simulink model "lane_departure"  (R2017a)
settings: Solver=FixedStepDiscrete  StartTime=0.0  StopTime=inf  FixedStep=1/25  RelTol=1e-3  EnableMultiTasking=on
libraries: visionsinks x1, dspvision x1, embdlinuxlib x1
settings Model: SimulationMode=external  Creator=ChiChaChai  LastModifiedBy=ChiChaChai
settings SolverCC: PositivePriorityOrder=on  AutoInsertRateTranBlk=on
settings OptimizationCC: UseFloatMulNetSlope=on  PassReuseOutputArgsAs=Individual arguments  ZeroExternalMemoryAtStartup=off  ZeroInternalMemoryAtStartup=off  NoFixptDivByZeroProtection=on  EfficientFloat2IntCast=on  LifeSpan=1  MaxStackSize=64
settings DebuggingCC: ParameterTunabilityLossMsg=error
settings HardwareCC: ProdBitPerPointer=32  ProdBitPerSizeT=32  ProdBitPerPtrDiffT=32  ProdLargestAtomicInteger=Long  ProdLargestAtomicFloat=Double  ProdWordSize=32  ProdHWDeviceType=ARM Compatible->ARM Cortex
settings SFSimCC: MATLABDynamicMemAlloc=off
settings RTWCC: SystemTargetFile=ert.tlc  HardwareBoard=Raspberry Pi  TLCOptions="-aInlineSetEventsForThisBaseRateFcn=TLC_FALSE -aSuppressMultiTaskScheduler=TLC_FALSE  -aRateBasedStepFcn=0"  TemplateMakefile=ert_default_tmf  Description=Embedded Coder  GenerateReport=on  Toolchain=GNU GCC Raspberry Pi  IncludeHyperlinkInReport=on  LaunchReport=on  GenerateTraceInfo=on  GenerateTraceReport=on  GenerateTraceReportSl=on  GenerateTraceReportSf=on  GenerateTraceReportEml=on  GenerateCodeMetricsReport=on
settings CodeAppCC: ForceParamTrailComments=on  IgnoreCustomStorageClasses=off  OperatorAnnotations=on  SimulinkDataObjDesc=on  SFDataObjDesc=on  MATLABFcnDesc=on  CustomSymbolStrGlobalVar=rt$N$M  CustomSymbolStrType=$N$M  CustomSymbolStrFcn=$N$M$F  CustomSymbolStrMacro=$N$M  InsertBlockDesc=on  MATLABSourceComments=on
settings ERTTargetCC: IncludeMdlTerminateFcn=off  CombineSignalStateStructs=on  SupportAbsoluteTime=off  SupportComplex=off  SupportNonInlinedSFcns=on  SupportVariableSizeSignals=on  ExtMode=on  ExtModeMexArgs='192.168.1.229' 0 17725  ERTFilePackagingFormat=CompactWithDataFile

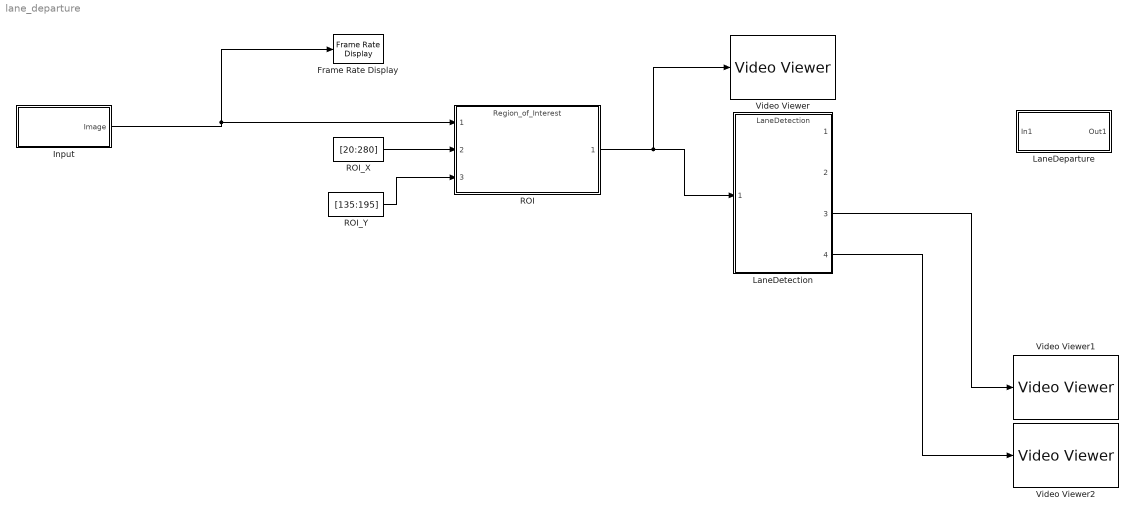
== system lane_departure ==
  Frame Rate Display : visionsinks/Frame Rate Display  UpdateRate=10
      settings: SourceProductName=Computer Vision System Toolbox  SourceProductBaseCode=VP
  "Input " : Subsystem
  LaneDeparture : Subsystem
  LaneDetection : ModelReference  ModelNameDialog=LaneDetection  SimulationMode=Normal  ModelReferenceVersion=1.110
  ROI : ModelReference  ModelNameDialog=Region_of_Interest  SimulationMode=Normal  ModelReferenceVersion=1.111
  ROI_X : Constant  Value=[20:280]
  ROI_Y : Constant  Value=[135:195]
  Video Viewer : VideoViewer  FigPos=[352.2 430 265.6 244.8]
  Video Viewer1 : VideoViewer  FigPos=[1078.6 490 417.6 304]
  Video Viewer2 : VideoViewer  FigPos=[633 490 417.6 304]
  wires:
  "Input "/1(Image) -> ROI/1, Frame Rate Display/1
  ROI_X/1 -> ROI/2
  ROI_Y/1 -> ROI/3
  ROI/1 -> LaneDetection/1, Video Viewer/1
  LaneDetection/3 -> Video Viewer1/1
  LaneDetection/4 -> Video Viewer2/1

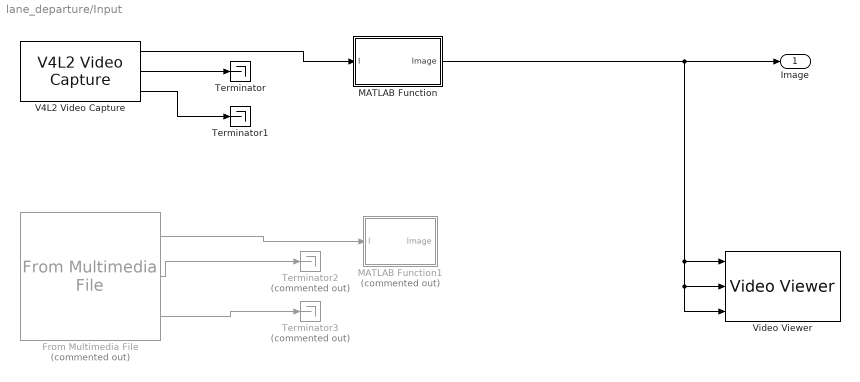
== system lane_departure/Input  ==
  From Multimedia File : dspvision/From Multimedia File  Commented=on  inputFilename=C:\Users\ChiChaChai\Documents\AMAS-2017\SelfDrivingCar_with_MATLAB\video.mp4  loop=on  numPlays=inf  outputStreams=Video only  videoDataType=uint8  audioDataType=int16  inheritSampleTime=off  userDefinedSampleTime=1/2  noAudioOutput=off  isIntensityVideo=off  fourcc=YCbCr 4:2:2  colorVideoFormat=One multidimensional signal  outputEOF=off  dataOrg=Column-major  audioFrameSize=1024  computeAudioFrameSize=off  outSamplingMode=Sample based
      settings: SourceProductBaseCode=VP
  MATLAB Function : MATLAB Function  TreatAsAtomicUnit=on
  MATLAB Function1 : MATLAB Function  Commented=on  TreatAsAtomicUnit=on
  Terminator : Terminator
  Terminator1 : Terminator
  Terminator2 : Terminator  Commented=on
  Terminator3 : Terminator  Commented=on
  V4L2 Video Capture : embdlinuxlib/V4L2 Video Capture  m_devName='/dev/video0'  roi=[0, 0, 640, 480]  imSizeSelection=320x240  imSize=[640, 480]  pixelFormat=YCbCr 4:2:2  pixelOrder=Planar  sampleTime=-1  simOutput=Colorbars  blockPlatform=Raspberry Pi
  Video Viewer : VideoViewer  imagePorts=separate color signals  FigPos=[13.8 430.8 317.6 247.2]
  Image : Outport
  wires:
  V4L2 Video Capture/2 -> Terminator/1
  V4L2 Video Capture/3 -> Terminator1/1
  V4L2 Video Capture/1 -> MATLAB Function/1(I)
  From Multimedia File/2 -> Terminator2/1
  From Multimedia File/3 -> Terminator3/1
  From Multimedia File/1 -> MATLAB Function1/1(I)
  MATLAB Function/1(Image) -> Video Viewer/2, Video Viewer/3, Video Viewer/1, Image/1

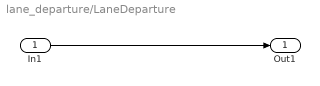
== system lane_departure/LaneDeparture ==
  In1 : Inport
  Out1 : Outport
  wires:
  In1/1 -> Out1/1

== matlab function lane_departure/Input /MATLAB Function1 ==
  data: I input; Image output
function Image = Flip(I)

Image = imrotate(I,180,'bilinear');

== matlab function lane_departure/Input /MATLAB Function ==
  data: I input; Image output
function Image = FlipAndRotate(I)
Image = imrotate(I,90,'bilinear');
Image = flip(Image,2);
